simulink model "partTwoThreeDifferentialDrive"  (R2021b)
settings: Solver=VariableStepAuto  StartTime=0.0  StopTime=10.0  RelTol=1e-3
settings Model: Creator=ericp  LastModifiedBy=ericp

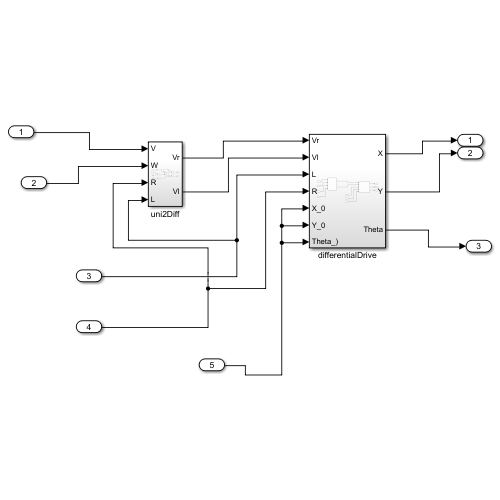
[thumbnail: Simulink's stored preview of the top-level diagram]
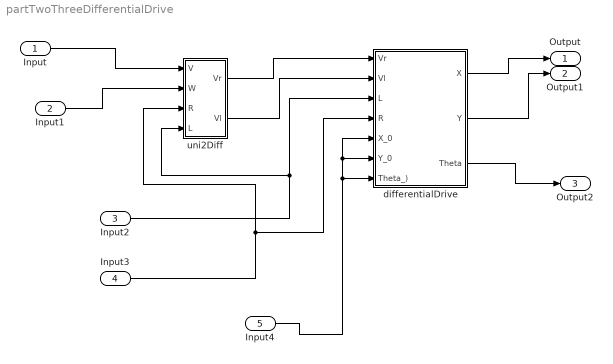
== system partTwoThreeDifferentialDrive ==
  Input : Inport
  Input1 : Inport  Port=2
  Input2 : Inport  Port=3
  Input3 : Inport  Port=4
  Input4 : Inport  Port=5
  differentialDrive : Subsystem
  uni2Diff : Subsystem
  Output : Outport
  Output1 : Outport  Port=2
  Output2 : Outport  Port=3
  wires:
  uni2Diff/1(Vr) -> differentialDrive/1(Vr)
  Input/1 -> uni2Diff/1(V)
  Input4/1 -> differentialDrive/6(Y_0), differentialDrive/5(X_0), differentialDrive/7(Theta_))
  Input3/1 -> uni2Diff/3(R), differentialDrive/4(R)
  Input1/1 -> uni2Diff/2(W)
  differentialDrive/3(Theta) -> Output2/1
  differentialDrive/1(X) -> Output/1
  uni2Diff/2(Vl) -> differentialDrive/2(Vl)
  Input2/1 -> uni2Diff/4(L), differentialDrive/3(L)
  differentialDrive/2(Y) -> Output1/1

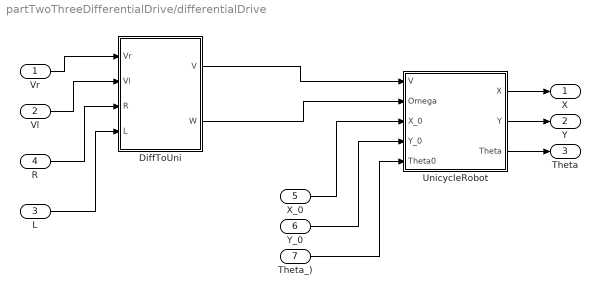
== system partTwoThreeDifferentialDrive/differentialDrive ==
  Vr : Inport
  Vl : Inport  Port=2
  L : Inport  Port=3
  R : Inport  Port=4
  X_0 : Inport  Port=5
  Y_0 : Inport  Port=6
  Theta_) : Inport  Port=7
  DiffToUni : Subsystem
  UnicycleRobot : Subsystem
  X : Outport
  Y : Outport  Port=2
  Theta : Outport  Port=3
  wires:
  Y_0/1 -> UnicycleRobot/4(Y_0)
  UnicycleRobot/3(Theta) -> Theta/1
  UnicycleRobot/1(X) -> X/1
  UnicycleRobot/2(Y) -> Y/1
  DiffToUni/1(V) -> UnicycleRobot/1(V)
  Theta_)/1 -> UnicycleRobot/5(Theta0)
  Vr/1 -> DiffToUni/1(Vr)
  DiffToUni/2(W) -> UnicycleRobot/2(Omega)
  R/1 -> DiffToUni/3(R)
  Vl/1 -> DiffToUni/2(Vl)
  L/1 -> DiffToUni/4(L)
  X_0/1 -> UnicycleRobot/3(X_0)

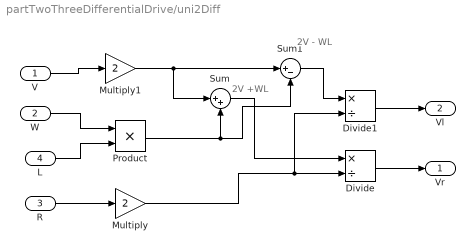
== system partTwoThreeDifferentialDrive/uni2Diff ==
  note: 2V +WL
  note: 2V - WL
  V : Inport
  W : Inport  Port=2
  R : Inport  Port=3
  L : Inport  Port=4
  Divide : Product  Inputs=*/
  Divide1 : Product  Inputs=*/
  Multiply : Gain  Gain=2
  Multiply1 : Gain  Gain=2
  Product : Product
  Sum : Sum  Inputs=|++
  Sum1 : Sum  Inputs=|+-
  Vr : Outport
  Vl : Outport  Port=2
  wires:
  V/1 -> Multiply1/1
  Divide/1 -> Vr/1
  Sum1/1 -> Divide1/1
  Multiply/1 -> Divide1/2, Divide/2
  Divide1/1 -> Vl/1
  L/1 -> Product/2
  R/1 -> Multiply/1
  Multiply1/1 -> Sum1/1, Sum/1
  Sum/1 -> Divide/1
  Product/1 -> Sum1/2, Sum/2
  W/1 -> Product/1

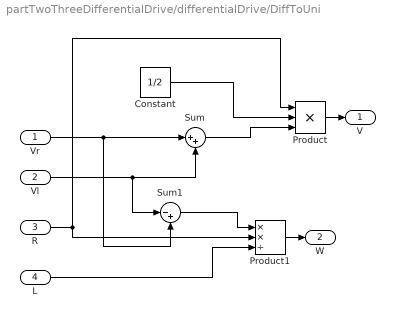
== system partTwoThreeDifferentialDrive/differentialDrive/DiffToUni ==
  Vr : Inport
  Vl : Inport  Port=2
  R : Inport  Port=3
  L : Inport  Port=4
  Constant : Constant  Value=1/2
  Product : Product  Inputs=3
  Product1 : Product  Inputs=**/  InputSameDT=on
  Sum : Sum  Inputs=|++
  Sum1 : Sum  Inputs=|-+
  V : Outport
  W : Outport  Port=2
  wires:
  Vl/1 -> Sum1/1, Sum/2
  L/1 -> Product1/3
  Sum/1 -> Product/3
  Vr/1 -> Sum1/2, Sum/1
  R/1 -> Product1/2, Product/1
  Constant/1 -> Product/2
  Sum1/1 -> Product1/1
  Product/1 -> V/1
  Product1/1 -> W/1

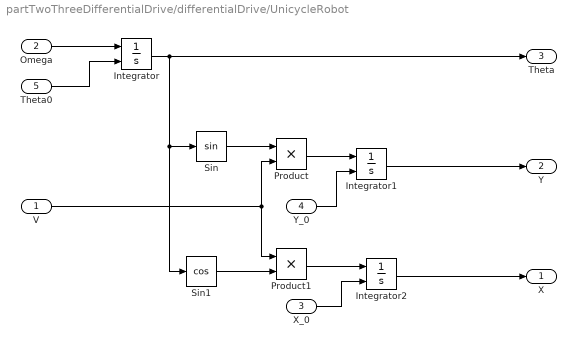
== system partTwoThreeDifferentialDrive/differentialDrive/UnicycleRobot ==
  V : Inport
  Omega : Inport  Port=2
  X_0 : Inport  Port=3
  Y_0 : Inport  Port=4
  Theta0 : Inport  Port=5
  Integrator : Integrator  InitialConditionSource=external
  Integrator1 : Integrator  InitialConditionSource=external
  Integrator2 : Integrator  InitialConditionSource=external
  Product : Product
  Product1 : Product
  Sin : Trigonometry
  Sin1 : Trigonometry  Operator=cos
  X : Outport
  Y : Outport  Port=2
  Theta : Outport  Port=3
  wires:
  Sin1/1 -> Product1/2
  V/1 -> Product1/1, Product/2
  Integrator/1 -> Theta/1, Sin1/1, Sin/1
  Integrator2/1 -> X/1
  Sin/1 -> Product/1
  Theta0/1 -> Integrator/2
  Y_0/1 -> Integrator1/2
  Omega/1 -> Integrator/1
  X_0/1 -> Integrator2/2
  Integrator1/1 -> Y/1
  Product1/1 -> Integrator2/1
  Product/1 -> Integrator1/1
